simulink model "dual500MHzPFB"  (Simulink 6.2)
settings: Solver=ode45  StartTime=0.0  StopTime=10000  RelTol=1e-3
libraries: xbsIndex_r3 x2070, casper_library x180, xps_library x12, gtkWave x5, gavrt_library x1
(part 10 of 20)

== system dual500MHzPFB/cfgspec/PFB_Subsystem/pfb_fir_real/pol1_in1_last_tap/pfb_real_add_tree ==
  din : Inport  Port=1  LatchInput=off
  sync : Inport  Port=2  LatchInput=off
  Reint0 : xbsIndex_r3/Reinterpret  force_arith_type=on  arith_type="Signed  (2's comp)"  force_bin_pt=on  bin_pt=CoeffBitWidth + BitWidthIn - 2  force_valid=on
  Reint1 : xbsIndex_r3/Reinterpret  force_arith_type=on  arith_type="Signed  (2's comp)"  force_bin_pt=on  bin_pt=CoeffBitWidth + BitWidthIn - 2  force_valid=on
  Slice0 : xbsIndex_r3/Slice  mode=Upper Bit Location + Width  nbits=CoeffBitWidth + BitWidthIn  bit1=-0*(CoeffBitWidth + BitWidthIn)  base1=MSB of Input  bit0=0  base0=MSB of Input  boolean_output=off  explicit_period=off  period=1  dbl_ovrd=off
  Slice1 : xbsIndex_r3/Slice  mode=Upper Bit Location + Width  nbits=CoeffBitWidth + BitWidthIn  bit1=-1*(CoeffBitWidth + BitWidthIn)  base1=MSB of Input  bit0=0  base0=MSB of Input  boolean_output=off  explicit_period=off  period=1  dbl_ovrd=off
  adder_tree1 : Subsystem  AncestorBlock=casper_library/Misc/adder_tree  mask(adder_tree){n_inputs=2, latency=2}
      mask prompts: n_inputs "Number of Inputs"; latency "Add Latency"
      mask help: Sums all inputs using a tree of adds and delays.
      mask init:
      | adder_tree_init(gcb, ...
      |     'n_inputs', n_inputs, ...
      |     'latency', latency);
      settings: AttributesFormatString=latency 2
      mask Help: eval('xlWeb([getenv(''MLIB_ROOT''), ''\doc\html\sp_adder_tree\sp_adder_tree.html''])')
  convert1 : xbsIndex_r3/Convert  arith_type="Signed  (2's comp)"  n_bits=BitWidthOut  bin_pt=BitWidthOut-1  quantization=Truncate  overflow=Saturate  latency=add_latency  explicit_period=off  period=1  dbl_ovrd=off  show_param=off  inserted_by_tool=off  pipeline=off
      settings: xl_area=[0, 0, 0, 0, 0, 0, 0]
  delay1 : xbsIndex_r3/Delay  latency=2  reg_retiming=off  explicit_period=off  period=1  en=off  accept_only_valid=off  init_zero=on  dbl_ovrd=off  show_param=off
      settings: xl_area=[0, 0, 0, 0, 0, 0, 0]
  scale1 : xbsIndex_r3/Scale  scale_factor=-2  explicit_period=off  period=1  dbl_ovrd=off
  dout : Outport
  sync_out : Outport  Port=2
  wires:
  adder_tree1/2(dout) -> scale1/1
  scale1/1 -> convert1/1
  convert1/1 -> dout/1
  sync/1 -> adder_tree1/1(sync)
  adder_tree1/1(sync_out) -> delay1/1
  delay1/1 -> sync_out/1
  din/1 -> Slice0/1, Slice1/1
  Slice0/1 -> Reint0/1
  Reint0/1 -> adder_tree1/2(din1)
  Slice1/1 -> Reint1/1
  Reint1/1 -> adder_tree1/3(din2)

== system dual500MHzPFB/cfgspec/PFB_Subsystem/pfb_fir_real/pol1_in2_first_tap/delay ==
  In1 : Inport  Port=1  LatchInput=off
  delay_bram : casper_library/Delays/delay_bram  DelayLen=2^(PFBSize-n_inputs)  bram_latency=bram_latency
  Out1 : Outport
  wires:
  In1/1 -> delay_bram/1
  delay_bram/1 -> Out1/1

== system dual500MHzPFB/cfgspec/PFB_Subsystem/pfb_fir_real/pol1_in2_first_tap/pfb_coeff_gen ==
  din : Inport  Port=1  LatchInput=off
  sync : Inport  Port=2  LatchInput=off
  Concat : xbsIndex_r3/Concat  num_inputs=2  explicit_period=off  period=1  dbl_ovrd=off
  Counter : xbsIndex_r3/Counter  cnt_type=Free Running  n_bits=8  bin_pt=0  arith_type=Unsigned  start_count=0  cnt_to=Inf  cnt_by_val=1  operation=Up  explicit_period=on  period=1  load_pin=off  rst=on  en=off  dbl_ovrd=off  show_param=off  use_rpm=on  gen_core=off
      settings: xl_area=[0, 0, 0, 0, 0, 0, 0]
  Delay : xbsIndex_r3/Delay  latency=bram_latency+1  reg_retiming=off  explicit_period=off  period=1  en=off  accept_only_valid=off  init_zero=on  dbl_ovrd=off  show_param=off
      settings: xl_area=[0, 0, 0, 0, 0, 0, 0]
  Delay1 : xbsIndex_r3/Delay  latency=3  reg_retiming=off  explicit_period=off  period=1  en=off  accept_only_valid=off  init_zero=on  dbl_ovrd=off  show_param=off
      settings: xl_area=[0, 0, 0, 0, 0, 0, 0]
  ROM1 : xbsIndex_r3/ROM  depth=256  initVector=[7.82033640873917e-005 0.000392792117321438 0.00071082554813207 0.00103311892199487 0.00136049907461725 0.00169380402655518 0.00203388258985642 0.00238159396690193 0.00273780734162119 0.00310340146326166 0.00347926422289714 0.00386629222286377 0.00426539033931678 0.00467747127810509 0.00510345512416486 0.00554426888463693 0.00600084602591724 0.00647412600485223 0.00696505379429587 0.00747457940324748 0.00800365739179369 0.00855324638108065 0.00912430855854599 0.00971780917864314 0.0103347160592936 0.0109759990743052 0.0116426296419981 0.0123355802102817 0.0130558237384286 0.0138043331757953 0.0145820809377384 0.0153900383789824 0.0162291752646908 0.0171004592395002 0.0180048552947743 0.0189433252343389 0.0199168271389599 0.0209263148298273 0.021972737331309 0.0230570383332419 0.0241801556530246 0.0253430206977808 0.0265465579268609 0.0277916843149512 0.0290793088160584 0.0304103318286413 0.0317856446621574 0.0332061290052946 0.0346726563961596 0.0361860876946888 0.0377472725575551 0.0393570489158354 0.0410162424557095 0.0427256661024564 0.0444861195080145 0.046298388542371 0.0481632447890453 0.0500814450449274 0.0520537308247352 0.0540808278703483 0.0561634456652778 0.0583022769545272 0.0604979972700995 0.0627512644624029 0.0650627182378034 0.067432979702574 0.0698626509134837 0.07235231443527 0.0749025329052334 0.0775138486051921 0.0801867830410294 0.082921836530065 0.0857194877964775 0.0885801935750023 0.0915043882231255 0.0944924833419901 0.0975448674062286 0.100661905402931 0.103843938479953 0.107091283603769 0.110404233227058 0.113783054966233 0.117227991289079 0.120739259212706 0.124317050011981 0.127961528938623 0.131672834951122 0.135451080455663 0.139296351058194 0.143208705327813 0.147188174571609 0.151234762621111 0.155348445630488 0.159529171886614 0.163776861631156 0.168091406894782 0.172472671343625 0.176920490138103 0.18143466980421 0.186014988117371 0.190661193998959 0.195373007425566 0.200150119351105 0.204992191641821 0.209898857024285 0.214869719046434 0.219904352051709 0.225002301166354 0.230163082299916 0.235386182158984 0.240671058274206 0.2460171390406 0.251423823771201 0.256890482764031 0.262416457382418 0.26800106014867 0.273643574851073 0.279343256664236 0.285099332282737 0.290911000068066 0.296777430208813 0.302697764894093 0.308671118500132 0.314696577789995 0.320773202126374 0.326900023697389 0.333076047755331 0.339300252868267 0.345571591184427 0.351888988709288 0.358251345595259 0.364657536443868 0.37110641062034 0.377596792580462 0.384127482209607 0.390697255173799 0.397304863282687 0.40394903486429 0.41062847515137 0.417341866679289 0.424087869695195 0.430865122578368 0.437672242271578 0.444507824723272 0.451370445340415 0.458258659451806 0.46517100278169 0.472105991933451 0.479062124883217 0.486037881483159 0.493031723974274 0.50004209750845 0.507067430679598 0.514106136063612 0.521156610766955 0.528217236983621 0.535286382560249 0.542362401569151 0.549443634889005 0.556528410792964 0.563615045543947 0.570701843996833 0.577787100207321 0.584869098047179 0.591946111825632 0.599016406916601 0.606078240391542 0.613129861657594 0.620169513100771 0.627195430733905 0.634205844849072 0.641198980674199 0.648173059033581 0.655126297012004 0.662056908622189 0.668963105475262 0.675843097453958 0.682695093388247 0.6895173017331 0.696307931248092 0.703065191678525 0.709787294437785 0.716472453290627 0.723118885037072 0.729724810196624 0.736288453692496 0.742808045535534 0.749281821507542 0.755708023843698 0.762084901913749 0.768410712901686 0.774683722483594 0.780902205503364 0.787064446645969 0.793168741108002 0.799213395265163 0.805196727336407 0.811117068044443 0.816972761272283 0.822762164715558 0.828483650530292 0.834135605975834 0.839716434052685 0.84522455413489 0.850658402596745 0.856016433433509 0.861297118875845 0.866498949997721 0.871620437317469 0.876660111391761 0.881616523402199 0.886488245734271 0.891273872548405 0.89597202034285 0.900581328508143 0.905100459872888 0.909528101240623 ...(+701 chars)]  arith_type="Signed  (2's comp)"  n_bits=8  bin_pt=7  latency=2  init_zero=on  explicit_period=off  period=1  rst=off  init_reg=0  en=off  dbl_ovrd=off  show_param=on  distributed_mem=off  use_rpm=on  gen_core=off
      settings: xl_area=[0, 0, 0, 0, 0, 0, 0]
  ROM2 : xbsIndex_r3/ROM  depth=256  initVector=[0.999993555614484 0.999895235614821 0.999677407720508 0.999340137306542 0.99888352558091 0.998307709543272 0.997612861929031 0.996799191138817 0.995866941153415 0.994816391434173 0.993647856808947 0.992361687343622 0.99095826819928 0.989438019475073 0.987801396036875 0.986048887331801 0.984181017188665 0.982198343604478 0.980101458517079 0.977890987564016 0.975567589827767 0.973131957567446 0.970584815937088 0.967926922690669 0.965159067873983 0.962282073503518 0.959296793232491 0.956204112004174 0.953004945692698 0.949700240731477 0.946290973729442 0.942778151075241 0.939162808529609 0.935446010806083 0.931628851140254 0.927712450847762 0.923697958871232 0.919586551316358 0.915379430977356 0.911077826851989 0.906682993646407 0.902196211270012 0.897618784320587 0.892952041559925 0.888197335380202 0.883356041261322 0.878429557219512 0.873419303247388 0.868326720745771 0.863153271947495 0.857900439333497 0.852569725041413 0.847162650267003 0.841680754658628 0.83612559570509 0.830498748117097 0.824801803202644 0.819036368236582 0.813204065824676 0.807306533262431 0.801345421888981 0.795322396436338 0.789239134374282 0.783097325251212 0.776898670031231 0.770644880427786 0.764337678234152 0.757978794651064 0.751569969611804 0.745112951105048 0.738609494495772 0.732061361844525 0.725470321225382 0.718838146042869 0.71216661434818 0.705457508154989 0.698712612755152 0.691933716034627 0.685122607789892 0.678281079045185 0.671410921370864 0.66451392620319 0.657591884165825 0.65064658439337 0.643679813857221 0.636693356694045 0.629688993537183 0.622668500851263 0.615633650270321 0.608586207939725 0.601527933862177 0.594460581248096 0.587385895870655 0.580305615425757 0.573221468897224 0.566135175927489 0.55904844619404 0.551962978791909 0.544880461622458 0.537802570788727 0.530730969997615 0.52366730996913 0.516613227852975 0.509570346652719 0.502540274657783 0.495524604883502 0.488524914519479 0.481542764386477 0.474579698402069 0.467637243055272 0.460716906890385 0.453820180000238 0.446948533529066 0.440103419185214 0.433286268763866 0.426498493679995 0.419741484511721 0.413016610554267 0.406325219384677 0.399668636437484 0.393048164591489 0.386465083767804 0.379920650539333 0.373416097751825 0.366952634156649 0.360531444055436 0.354153686956706 0.347820497244626 0.34153298386 0.335292229993622 0.329099292792089 0.322955203076182 0.316860965071917 0.310817556154338 0.304825926604156 0.2988869993773 0.293001669887455 0.287170805801649 0.281395246848952 0.275675804642333 0.270013262513728 0.264408375362351 0.258861869516288 0.253374442607394 0.247946763459516 0.242579471990057 0.237273179124887 0.232028466726598 0.226845887536105 0.221725965127573 0.21666919387666 0.211676038942041 0.206746936260191 0.201882292553387 0.197082485350882 0.192347863023202 0.187678744829518 0.183075420978016 0.178538152699211 0.174067172332122 0.169662683423225 0.165324860838114 0.161053850885749 0.156849771455227 0.152712712164937 0.148642734524024 0.144639872106008 0.14070413073448 0.136835488680706 0.133033896873036 0.129299279117972 0.125631532332744 0.12203052678926 0.118496106369262 0.115028088830537 0.111626266084031 0.108290404481666 0.105020245114723 0.101815504122587 0.0986758730116877 0.0956010189844369 0.0925905852779795 0.0896441915125591 0.0867614340492978 0.0839418863571882 0.0811850993890874 0.0784906019665026 0.0758579011729519 0.0732864827556818 0.0707758115355173 0.0683253318246198 0.0659344678519223 0.0636026241960095 0.0613291862252073 0.0591135205446423 0.056954975450031 0.0548528813879534 0.0528065514223651 0.0508152817070987 0.0488783519641021 0.0469950259671621 0.0451645520308558 0.0433861635044739 0.0416590792706549 0.0399825042484717 0.0383556299007058 0.0367776347450473 0.0352476848689546 0.0337649344479084 0.0323285262667932 0.0309375922441371 0.029591253958944 0.0282886231798464 0.0270288023963116 0.0258108853516301 0.0246339575774173 0.0234970969293587 0.0223993741239277 0.0213398532758088 0.0203175924357544 ...(+708 chars)]  arith_type="Signed  (2's comp)"  n_bits=8  bin_pt=7  latency=2  init_zero=on  explicit_period=off  period=1  rst=off  init_reg=0  en=off  dbl_ovrd=off  show_param=on  distributed_mem=off  use_rpm=on  gen_core=off
      settings: xl_area=[0, 0, 0, 0, 0, 0, 0]
  Register : xbsIndex_r3/Register  init=0  reg_only_valid=off  explicit_period=off  period=1  rst=off  en=off  out_en=off  dbl_ovrd=off  show_param=off
      settings: xl_area=[0, 0, 0, 0, 0, 0, 0]
  Reinterpret1 : xbsIndex_r3/Reinterpret  force_arith_type=on  arith_type=Unsigned  force_bin_pt=on  bin_pt=0  force_valid=on
  Reinterpret2 : xbsIndex_r3/Reinterpret  force_arith_type=on  arith_type=Unsigned  force_bin_pt=on  bin_pt=0  force_valid=on
  dout : Outport
  sync_out : Outport  Port=2
  coeff : Outport  Port=3
  wires:
  din/1 -> Delay1/1
  Delay1/1 -> dout/1
  sync/1 -> Counter/1, Delay/1
  Delay/1 -> sync_out/1
  Concat/1 -> Register/1
  Register/1 -> coeff/1
  Counter/1 -> ROM1/1, ROM2/1
  ROM1/1 -> Reinterpret1/1
  Reinterpret1/1 -> Concat/1
  ROM2/1 -> Reinterpret2/1
  Reinterpret2/1 -> Concat/2

== system dual500MHzPFB/cfgspec/PFB_Subsystem/pfb_fir_real/pol1_in2_last_tap/pfb_real_add_tree ==
  din : Inport  Port=1  LatchInput=off
  sync : Inport  Port=2  LatchInput=off
  Reint0 : xbsIndex_r3/Reinterpret  force_arith_type=on  arith_type="Signed  (2's comp)"  force_bin_pt=on  bin_pt=CoeffBitWidth + BitWidthIn - 2  force_valid=on
  Reint1 : xbsIndex_r3/Reinterpret  force_arith_type=on  arith_type="Signed  (2's comp)"  force_bin_pt=on  bin_pt=CoeffBitWidth + BitWidthIn - 2  force_valid=on
  Slice0 : xbsIndex_r3/Slice  mode=Upper Bit Location + Width  nbits=CoeffBitWidth + BitWidthIn  bit1=-0*(CoeffBitWidth + BitWidthIn)  base1=MSB of Input  bit0=0  base0=MSB of Input  boolean_output=off  explicit_period=off  period=1  dbl_ovrd=off
  Slice1 : xbsIndex_r3/Slice  mode=Upper Bit Location + Width  nbits=CoeffBitWidth + BitWidthIn  bit1=-1*(CoeffBitWidth + BitWidthIn)  base1=MSB of Input  bit0=0  base0=MSB of Input  boolean_output=off  explicit_period=off  period=1  dbl_ovrd=off
  adder_tree1 : Subsystem  AncestorBlock=casper_library/Misc/adder_tree  mask(adder_tree){n_inputs=2, latency=2}
      mask prompts: n_inputs "Number of Inputs"; latency "Add Latency"
      mask help: Sums all inputs using a tree of adds and delays.
      mask init:
      | adder_tree_init(gcb, ...
      |     'n_inputs', n_inputs, ...
      |     'latency', latency);
      settings: AttributesFormatString=latency 2
      mask Help: eval('xlWeb([getenv(''MLIB_ROOT''), ''\doc\html\sp_adder_tree\sp_adder_tree.html''])')
  convert1 : xbsIndex_r3/Convert  arith_type="Signed  (2's comp)"  n_bits=BitWidthOut  bin_pt=BitWidthOut-1  quantization=Truncate  overflow=Saturate  latency=add_latency  explicit_period=off  period=1  dbl_ovrd=off  show_param=off  inserted_by_tool=off  pipeline=off
      settings: xl_area=[0, 0, 0, 0, 0, 0, 0]
  delay1 : xbsIndex_r3/Delay  latency=2  reg_retiming=off  explicit_period=off  period=1  en=off  accept_only_valid=off  init_zero=on  dbl_ovrd=off  show_param=off
      settings: xl_area=[0, 0, 0, 0, 0, 0, 0]
  scale1 : xbsIndex_r3/Scale  scale_factor=-2  explicit_period=off  period=1  dbl_ovrd=off
  dout : Outport
  sync_out : Outport  Port=2
  wires:
  adder_tree1/2(dout) -> scale1/1
  scale1/1 -> convert1/1
  convert1/1 -> dout/1
  sync/1 -> adder_tree1/1(sync)
  adder_tree1/1(sync_out) -> delay1/1
  delay1/1 -> sync_out/1
  din/1 -> Slice0/1, Slice1/1
  Slice0/1 -> Reint0/1
  Reint0/1 -> adder_tree1/2(din1)
  Slice1/1 -> Reint1/1
  Reint1/1 -> adder_tree1/3(din2)

== system dual500MHzPFB/cfgspec/PFB_Subsystem/pfb_fir_real/pol1_in3_first_tap/delay ==
  In1 : Inport  Port=1  LatchInput=off
  delay_bram : casper_library/Delays/delay_bram  DelayLen=2^(PFBSize-n_inputs)  bram_latency=bram_latency
  Out1 : Outport
  wires:
  In1/1 -> delay_bram/1
  delay_bram/1 -> Out1/1

== system dual500MHzPFB/cfgspec/PFB_Subsystem/pfb_fir_real/pol1_in3_first_tap/pfb_coeff_gen ==
  din : Inport  Port=1  LatchInput=off
  sync : Inport  Port=2  LatchInput=off
  Concat : xbsIndex_r3/Concat  num_inputs=2  explicit_period=off  period=1  dbl_ovrd=off
  Counter : xbsIndex_r3/Counter  cnt_type=Free Running  n_bits=8  bin_pt=0  arith_type=Unsigned  start_count=0  cnt_to=Inf  cnt_by_val=1  operation=Up  explicit_period=on  period=1  load_pin=off  rst=on  en=off  dbl_ovrd=off  show_param=off  use_rpm=on  gen_core=off
      settings: xl_area=[0, 0, 0, 0, 0, 0, 0]
  Delay : xbsIndex_r3/Delay  latency=bram_latency+1  reg_retiming=off  explicit_period=off  period=1  en=off  accept_only_valid=off  init_zero=on  dbl_ovrd=off  show_param=off
      settings: xl_area=[0, 0, 0, 0, 0, 0, 0]
  Delay1 : xbsIndex_r3/Delay  latency=3  reg_retiming=off  explicit_period=off  period=1  en=off  accept_only_valid=off  init_zero=on  dbl_ovrd=off  show_param=off
      settings: xl_area=[0, 0, 0, 0, 0, 0, 0]
  ROM1 : xbsIndex_r3/ROM  depth=256  initVector=[0.000156571753004131 0.000471945891501983 0.000790967418464927 0.00111445452761384 0.00144323688731232 0.0017781552531742 0.00212006107274008 0.0024698160823956 0.00282829189670815 0.00319636959036365 0.00357493927288892 0.00396489965634961 0.00436715761621773 0.00478262774560706 0.00521223190307826 0.00565689875421988 0.00611756330721485 0.006595166442606 0.0070906544374775 0.00760497848427273 0.00813909420447243 0.00869396115736018 0.00927054234410557 0.00986980370739833 0.0104927136268696 0.0111402424105394 0.0118133617825326 0.0125130443673066 0.0132402631706387 0.013995991057622 0.0147812002279213 0.0155968616885416 0.016443944724367 0.0173234163667243 0.0182362408602338 0.0191833791282049 0.0201657882368408 0.0211844208585156 0.0222402247343869 0.0233341421366126 0.0244671093304362 0.0256400560364093 0.0268539048930204 0.028109570919997 0.0294079609825521 0.0307499732568442 0.0321364966969199 0.0335684105034094 0.0350465835942454 0.0365718740776727 0.03814512872782 0.0397671824631001 0.0414388578277084 0.0431609644764848 0.0449342986634068 0.0467596427339775 0.0486377646217729 0.0505694173494113 0.0525553385342047 0.0545962498987528 0.0566928567867364 0.0588458476841667 0.0610558937463428 0.0633236483307712 0.0656497465362942 0.0680348047486762 0.0704794201928911 0.0729841704923531 0.0755496132353287 0.0781762855487681 0.080864703679787 0.0836153625850295 0.0864287355281387 0.0893052736855576 0.0922454057608818 0.0952495376079764 0.0983180518630736 0.101451307586057 0.104649639911135 0.107913359707113 0.111242753247444 0.114638081890267 0.118099581768609 0.121627463490941 0.125221911852256 0.128883085555861 0.132611116946024 0.136406111751676 0.140268148841289 0.144197279989117 0.148193529652922 0.152256894763353 0.156387344525091 0.160584820229917 0.164849235081815 0.169180474034232 0.173578393639624 0.178042821911379 0.182573558198244 0.187170373071336 0.191833008223839 0.196561176383476 0.201354561237828 0.206212817372591 0.211135570222817 0.216122416037231 0.22117292185565 0.226286625499582 0.231463035576027 0.236701631494537 0.242001863497553 0.247363152704048 0.252784891166504 0.258266441941216 0.263807139171958 0.269406288186976 0.275063165609337 0.280777019480592 0.286547069397754 0.292372506663552 0.298252494449934 0.304186167974785 0.310172634691807 0.316210974493512 0.322300239927273 0.328439456424369 0.334627622541945 0.340863710217824 0.347146665038078 0.353475406517269 0.359848828391271 0.36626579892256 0.372725161217884 0.379225733558168 0.385766309740569 0.392345659432526 0.398962528537691 0.405615639573596 0.412303692060908 0.419025362924137 0.425779306903621 0.432564156978649 0.439378524801535 0.446221001142489 0.453090156345094 0.459984540792213 0.466902685382136 0.473843102014779 0.48080428408772 0.487784707001898 0.49478282867673 0.501797090074468 0.508825915733558 0.515867714310774 0.522920879131923 0.529983788750869 0.537054807516645 0.54413228614842 0.551214562318069 0.558299961240106 0.565386796268718 0.572473369501655 0.579557972390709 0.586638886358525 0.593714383421474 0.600782726818319 0.607842171644411 0.614890965491117 0.62192734909023 0.628949556963061 0.635955818073934 0.642944356487798 0.649913392031675 0.656861140959638 0.663785816621042 0.670685630131702 0.677558791047733 0.684403508041737 0.691217989581062 0.698000444607801 0.704749083220269 0.711462117355605 0.718137761473247 0.724774233238938 0.731369754208968 0.737922550514358 0.744430853544664 0.750892900631098 0.757306935728673 0.763671210097042 0.769983982979752 0.776243522281579 0.782448105243668 0.788596019116149 0.794685561827938 0.800715042653424 0.806682782875726 0.812587116446239 0.818426390640147 0.824198966707636 0.829903220520478 0.835537543213724 0.84110034182219 0.846590039911459 0.852005078203117 0.85734391519392 0.862605027768629 0.867786911806227 0.872888082779229 0.87790707634584 0.88284244893466 0.887692778321693 0.892456664199373 0.897132728737377 0.901719617134936 0.90621599816441 0.910620564705884 ...(+696 chars)]  arith_type="Signed  (2's comp)"  n_bits=8  bin_pt=7  latency=2  init_zero=on  explicit_period=off  period=1  rst=off  init_reg=0  en=off  dbl_ovrd=off  show_param=on  distributed_mem=off  use_rpm=on  gen_core=off
      settings: xl_area=[0, 0, 0, 0, 0, 0, 0]
  ROM2 : xbsIndex_r3/ROM  depth=256  initVector=[0.999980181706812 0.999851980565338 0.999604284511911 0.999237167882849 0.998750740838502 0.998145149318279 0.99742057498107 0.996577235131088 0.995615382629159 0.994535305789518 0.993337328262134 0.99202180890064 0.990589141615924 0.989039755215435 0.987374113228298 0.985592713716306 0.983696089070883 0.981684805796099 0.979559464277863 0.97732069853937 0.974969175982937 0.972505597118337 0.969930695277763 0.967245236317542 0.96445001830675 0.961545871202867 0.958533656514614 0.955414266952141 0.952188626064713 0.948857687866076 0.945422436447659 0.941883885579808 0.938243078301218 0.934501086496762 0.93065901046392 0.926717978467979 0.922679146286243 0.918543696741437 0.914312839224529 0.909987809207196 0.905569867744142 0.901060300965507 0.896460419559603 0.891771558246203 0.886995075240635 0.882132351708915 0.877184791214188 0.872153819154706 0.867040882193617 0.86184744768082 0.856575003067155 0.851225055311182 0.845799130278843 0.840298772136253 0.83472554273592 0.829081020996665 0.823366802277519 0.817584497745891 0.811735733740289 0.805822151127884 0.799845404657212 0.793807162306308 0.787709104626554 0.781552924082562 0.775340324388371 0.76907301984027 0.762752734646535 0.756381202254406 0.749960164674578 0.743491371803535 0.736976580744021 0.730417555123955 0.723816064414095 0.71717388324476 0.710492790721915 0.703774569742931 0.697021006312307 0.690233888857689 0.683415007546466 0.676566153603261 0.669689118628614 0.662785693919171 0.655857669789663 0.648906834896993 0.641934975566721 0.634943875122243 0.627935313216969 0.620911065169787 0.613872901304108 0.606822586290777 0.599761878495151 0.592692529328615 0.585616282604827 0.578534873900973 0.571450029924306 0.56436346788425 0.557276894870328 0.550192007236204 0.543110489990084 0.536034016191747 0.528964246356468 0.521902827866082 0.514851394387443 0.507811565298521 0.500784945122391 0.493773122969342 0.486777671987345 0.479800148821113 0.472842093079979 0.465905026814805 0.458990454004159 0.452099860049946 0.445234711282726 0.438396454476901 0.431586516375986 0.424806303228137 0.418057200332153 0.411340571594091 0.40465775909472 0.398010082667942 0.391398839490374 0.384825303682239 0.378290725919721 0.371796333058942 0.365343327771685 0.358932888193021 0.352566167580962 0.34624429398826 0.33996836994648 0.333739472162456 0.32755865122724 0.321426931337641 0.31534531003045 0.309314757929439 0.303336218505222 0.297410607848047 0.291538814453586 0.2857216990218 0.279960094268917 0.274254804752596 0.268606606710293 0.263016247910897 0.257484447519645 0.252011895976347 0.246599254886948 0.241247156928422 0.235956205767024 0.230726975989882 0.225560013049927 0.220455833224157 0.215414923585196 0.210437741986143 0.205524717058656 0.20067624822426 0.195892705718796 0.191174430630003 0.18652173494814 0.181934901629597 0.177414184673436 0.172959809210765 0.168571971606878 0.164250839576072 0.159996552309034 0.155809220612716 0.151688927062585 0.147635726167125 0.143649644544501 0.139730681111232 0.135878807282765 0.132093967185811 0.128376077882305 0.124725029604834 0.121140686003409 0.117622884403397 0.114171436074477 0.110786126510436 0.107466715719658 0.104212938526102 0.101024504880621 0.0979011001824149 0.0948423856104419 0.0918479984645913 0.088917552516421 0.0860506383692603 0.083246823827471 0.0805056542746607 0.0778266530606313 0.0752093218968506 0.0726531412602235 0.0701575708049404 0.0677220497821762 0.0653459974674089 0.0630288135951235 0.0607698788006672 0.0585685550690139 0.0564241861901975 0.054336098221168 0.0523035999538251 0.0503259833889764 0.048402524215972 0.0465324822977585 0.0447151021610977 0.0429496134916917 0.0412352316339554 0.0395711580951738 0.0379565810537831 0.0363906758715103 0.0348726056091064 0.0334015215454071 0.0319765636994546 0.0305968613554102 0.0292615335899919 0.0279696898021663 0.0267204302448249 0.0255128465581769 0.0243460223045864 0.0232190335045865 0.0221309491737983 0.0210808318604881 0.0200677381834912 0.0190907193702359 ...(+687 chars)]  arith_type="Signed  (2's comp)"  n_bits=8  bin_pt=7  latency=2  init_zero=on  explicit_period=off  period=1  rst=off  init_reg=0  en=off  dbl_ovrd=off  show_param=on  distributed_mem=off  use_rpm=on  gen_core=off
      settings: xl_area=[0, 0, 0, 0, 0, 0, 0]
  Register : xbsIndex_r3/Register  init=0  reg_only_valid=off  explicit_period=off  period=1  rst=off  en=off  out_en=off  dbl_ovrd=off  show_param=off
      settings: xl_area=[0, 0, 0, 0, 0, 0, 0]
  Reinterpret1 : xbsIndex_r3/Reinterpret  force_arith_type=on  arith_type=Unsigned  force_bin_pt=on  bin_pt=0  force_valid=on
  Reinterpret2 : xbsIndex_r3/Reinterpret  force_arith_type=on  arith_type=Unsigned  force_bin_pt=on  bin_pt=0  force_valid=on
  dout : Outport
  sync_out : Outport  Port=2
  coeff : Outport  Port=3
  wires:
  din/1 -> Delay1/1
  Delay1/1 -> dout/1
  sync/1 -> Counter/1, Delay/1
  Delay/1 -> sync_out/1
  Concat/1 -> Register/1
  Register/1 -> coeff/1
  Counter/1 -> ROM1/1, ROM2/1
  ROM1/1 -> Reinterpret1/1
  Reinterpret1/1 -> Concat/1
  ROM2/1 -> Reinterpret2/1
  Reinterpret2/1 -> Concat/2

== system dual500MHzPFB/cfgspec/PFB_Subsystem/pfb_fir_real/pol1_in3_last_tap/pfb_real_add_tree ==
  din : Inport  Port=1  LatchInput=off
  sync : Inport  Port=2  LatchInput=off
  Reint0 : xbsIndex_r3/Reinterpret  force_arith_type=on  arith_type="Signed  (2's comp)"  force_bin_pt=on  bin_pt=CoeffBitWidth + BitWidthIn - 2  force_valid=on
  Reint1 : xbsIndex_r3/Reinterpret  force_arith_type=on  arith_type="Signed  (2's comp)"  force_bin_pt=on  bin_pt=CoeffBitWidth + BitWidthIn - 2  force_valid=on
  Slice0 : xbsIndex_r3/Slice  mode=Upper Bit Location + Width  nbits=CoeffBitWidth + BitWidthIn  bit1=-0*(CoeffBitWidth + BitWidthIn)  base1=MSB of Input  bit0=0  base0=MSB of Input  boolean_output=off  explicit_period=off  period=1  dbl_ovrd=off
  Slice1 : xbsIndex_r3/Slice  mode=Upper Bit Location + Width  nbits=CoeffBitWidth + BitWidthIn  bit1=-1*(CoeffBitWidth + BitWidthIn)  base1=MSB of Input  bit0=0  base0=MSB of Input  boolean_output=off  explicit_period=off  period=1  dbl_ovrd=off
  adder_tree1 : Subsystem  AncestorBlock=casper_library/Misc/adder_tree  mask(adder_tree){n_inputs=2, latency=2}
      mask prompts: n_inputs "Number of Inputs"; latency "Add Latency"
      mask help: Sums all inputs using a tree of adds and delays.
      mask init:
      | adder_tree_init(gcb, ...
      |     'n_inputs', n_inputs, ...
      |     'latency', latency);
      settings: AttributesFormatString=latency 2
      mask Help: eval('xlWeb([getenv(''MLIB_ROOT''), ''\doc\html\sp_adder_tree\sp_adder_tree.html''])')
  convert1 : xbsIndex_r3/Convert  arith_type="Signed  (2's comp)"  n_bits=BitWidthOut  bin_pt=BitWidthOut-1  quantization=Truncate  overflow=Saturate  latency=add_latency  explicit_period=off  period=1  dbl_ovrd=off  show_param=off  inserted_by_tool=off  pipeline=off
      settings: xl_area=[0, 0, 0, 0, 0, 0, 0]
  delay1 : xbsIndex_r3/Delay  latency=2  reg_retiming=off  explicit_period=off  period=1  en=off  accept_only_valid=off  init_zero=on  dbl_ovrd=off  show_param=off
      settings: xl_area=[0, 0, 0, 0, 0, 0, 0]
  scale1 : xbsIndex_r3/Scale  scale_factor=-2  explicit_period=off  period=1  dbl_ovrd=off
  dout : Outport
  sync_out : Outport  Port=2
  wires:
  adder_tree1/2(dout) -> scale1/1
  scale1/1 -> convert1/1
  convert1/1 -> dout/1
  sync/1 -> adder_tree1/1(sync)
  adder_tree1/1(sync_out) -> delay1/1
  delay1/1 -> sync_out/1
  din/1 -> Slice0/1, Slice1/1
  Slice0/1 -> Reint0/1
  Reint0/1 -> adder_tree1/2(din1)
  Slice1/1 -> Reint1/1
  Reint1/1 -> adder_tree1/3(din2)

== system dual500MHzPFB/cfgspec/PFB_Subsystem/pfb_fir_real/pol1_in4_first_tap/delay ==
  In1 : Inport  Port=1  LatchInput=off
  delay_bram : casper_library/Delays/delay_bram  DelayLen=2^(PFBSize-n_inputs)  bram_latency=bram_latency
  Out1 : Outport
  wires:
  In1/1 -> delay_bram/1
  delay_bram/1 -> Out1/1

== system dual500MHzPFB/cfgspec/PFB_Subsystem/pfb_fir_real/pol1_in4_first_tap/pfb_coeff_gen ==
  din : Inport  Port=1  LatchInput=off
  sync : Inport  Port=2  LatchInput=off
  Concat : xbsIndex_r3/Concat  num_inputs=2  explicit_period=off  period=1  dbl_ovrd=off
  Counter : xbsIndex_r3/Counter  cnt_type=Free Running  n_bits=8  bin_pt=0  arith_type=Unsigned  start_count=0  cnt_to=Inf  cnt_by_val=1  operation=Up  explicit_period=on  period=1  load_pin=off  rst=on  en=off  dbl_ovrd=off  show_param=off  use_rpm=on  gen_core=off
      settings: xl_area=[0, 0, 0, 0, 0, 0, 0]
  Delay : xbsIndex_r3/Delay  latency=bram_latency+1  reg_retiming=off  explicit_period=off  period=1  en=off  accept_only_valid=off  init_zero=on  dbl_ovrd=off  show_param=off
      settings: xl_area=[0, 0, 0, 0, 0, 0, 0]
  Delay1 : xbsIndex_r3/Delay  latency=3  reg_retiming=off  explicit_period=off  period=1  en=off  accept_only_valid=off  init_zero=on  dbl_ovrd=off  show_param=off
      settings: xl_area=[0, 0, 0, 0, 0, 0, 0]
  ROM1 : xbsIndex_r3/ROM  depth=256  initVector=[0.000235117647765776 0.000551327569575741 0.000871388331650675 0.00119612103225011 0.00152635814818096 0.00186294314540636 0.0022067300817663 0.00255858320198372 0.00291937652513412 0.00328999342476105 0.00367132620182454 0.00406427565067298 0.00446975061823393 0.00488866755662283 0.00532195006937266 0.00577052845149145 0.00623533922355848 0.00671732466007321 0.00721743231227507 0.00773661452565523 0.00827582795238525 0.00883603305889021 0.00941819362879768 0.0100232762614963 0.0106522498665412 0.0113060851541457 0.0119857541220021 0.0126922295386765 0.0134264844238244 0.0141894915254781 0.0149822227946568 0.0158056488575538 0.0166607384855574 0.017548458063362 0.0184697710554301 0.0194256374710662 0.0204170133283646 0.0214448501172952 0.0225100942621926 0.0236136865839149 0.0247565617619379 0.0259396477966543 0.0271638654721455 0.0284301278196944 0.0297393395823103 0.031092396680534 0.0324901856797932 0.0339335832595792 0.0354234556847124 0.0369606582789679 0.0385460349013288 0.0401804174251365 0.0418646252204042 0.0435994646395624 0.0453857285069007 0.0472241956119709 0.0491156302072151 0.0510607815100817 0.0530603832098875 0.0551151529796884 0.0572257919934118 0.0593929844485101 0.0616173970943848 0.0638996787668347 0.0662404599287766 0.0686403522174832 0.071099947998584 0.0736198199270695 0.0762005205155353 0.0788425817099054 0.0815465144728618 0.0843128083752139 0.0871419311954306 0.0900343285275589 0.092990423397747 0.0960106158895877 0.0990952827784922 0.102244777175303 0.105459428179349 0.108739540541143 0.112085394334912 0.115497244641159 0.118975321239438 0.12251982831152 0.126130944155138 0.129808820908474 0.133553584285556 0.13736533332274 0.141244140136412 0.145190049692087 0.149203079585039 0.153283219832602 0.157430432678291 0.161644652407862 0.165925785177441 0.170273708853853 0.174688272867243 0.179169298076123 0.183716576644931 0.188329871934205 0.193008918403472 0.197753421526913 0.202563057721923 0.207437474290597 0.212376289374241 0.217379091920954 0.222445441666344 0.227574869127416 0.232766875609693 0.238020933227584 0.243336484938052 0.248712944587585 0.254149696972505 0.259646097912613 0.265201474338185 0.270815124390307 0.276486317534554 0.282214294687982 0.287998268359427 0.293837422803077 0.299730914185284 0.305677870764572 0.311677393084804 0.317728554181443 0.323830399800861 0.329981948632614 0.336182192554631 0.342430096891214 0.348724600683793 0.355064616974316 0.361449033101202 0.367876711007733 0.374346487562795 0.380857174893835 0.38740756073192 0.393996408768776 0.400622459025663 0.407284428233955 0.41398101022727 0.420710876345013 0.427472675847161 0.434265036340141 0.441086564213617 0.44793584508803 0.454811444272702 0.461711907234316 0.468635760075602 0.475581510024006 0.482547645930165 0.489532638775981 0.496534942192067 0.503552992984374 0.510585211669765 0.517630003020315 0.524685756616119 0.531750847406352 0.538823636278379 0.545902470634637 0.552985684977073 0.560071601498875 0.567158530683245 0.574244771908958 0.581328614062453 0.588408336156179 0.59548220795295 0.60254849059601 0.609605437244566 0.616651293714493 0.623684299123933 0.63070268654352 0.637704683650928 0.644688513389471 0.651652394630459 0.65859454283902 0.665513170743091 0.672406489005293 0.679272706897384 0.686110032976994 0.692916675766342 0.699690844432641 0.706430749469876 0.713134603381663 0.719800621364874 0.726427021993738 0.733012027904095 0.739553866477515 0.746050770524958 0.752500978969682 0.758902737529087 0.76525429939519 0.771553925913424 0.777799887259458 0.783990463113728 0.790123943333386 0.796198628621342 0.802212831192126 0.808164875434248 0.814053098568757 0.819875851303714 0.825631498484268 0.831318419738052 0.836935010115596 0.842479680725471 0.84795085936388 0.853346991138395 0.858666539085575 0.863907984782168 0.869069828949628 0.874150592051666 0.879148814884566 0.884063059159991 0.888891908080022 0.893633966904157 0.898287863508018 0.902852248933504 0.907325797930147 0.911707209487413 ...(+699 chars)]  arith_type="Signed  (2's comp)"  n_bits=8  bin_pt=7  latency=2  init_zero=on  explicit_period=off  period=1  rst=off  init_reg=0  en=off  dbl_ovrd=off  show_param=on  distributed_mem=off  use_rpm=on  gen_core=off
      settings: xl_area=[0, 0, 0, 0, 0, 0, 0]
  ROM2 : xbsIndex_r3/ROM  depth=256  initVector=[0.999959336786865 0.999801256908778 0.999523697342405 0.999126741383489 0.998610508141931 0.997975152493165 0.997220865014935 0.99634787190949 0.99535643491125 0.994246851179977 0.993019453179501 0.991674608542054 0.990212719918283 0.988634224813006 0.986939595406783 0.985129338363398 0.983203994623318 0.981164139183251 0.979010380861888 0.976743362051936 0.974363758458571 0.971872278824412 0.969269664641163 0.96655668984804 0.963734160517132 0.960802914525833 0.957763821216508 0.954617781043538 0.951365725207906 0.948008615279514 0.944547442807368 0.940983228917847 0.937317023901219 0.933549906786599 0.92968298490555 0.92571739344452 0.921654294986329 0.917494879040905 0.913240361565502 0.908891984474602 0.904451015139734 0.899918745879451 0.895296493439671 0.890585598464651 0.885787424958816 0.880903359739698 0.875934811882229 0.870883212154659 0.865750012446327 0.860536685187583 0.855244722762093 0.849875636911818 0.844430958134928 0.838912235076933 0.833321033915289 0.827658937737797 0.821927545915033 0.816128473467133 0.810263350425193 0.804333821187595 0.798341543871533 0.792288189660053 0.78617544214488 0.780004996665351 0.773778559643742 0.767497847917287 0.761164588067204 0.754780515745012 0.748347374996464 0.741866917583381 0.735340902303706 0.72877109431008 0.722159264427236 0.715507188468543 0.70881664655197 0.702089422415814 0.695327302734468 0.688532076434552 0.681705534011708 0.674849466848357 0.667965666532734 0.661055924179494 0.654122029752188 0.647165771387927 0.640188934724505 0.633193302230307 0.62618065253728 0.619152759777259 0.612111392921958 0.605058315126893 0.597995283079545 0.590924046352026 0.583846346758558 0.576763917718018 0.569678483621844 0.562591759207569 0.555505448938255 0.548421246388095 0.541340833634453 0.53426588065659 0.527198044741348 0.520138969896043 0.513090286268806 0.506053609576635 0.499030540541388 0.492022664333961 0.485031550026882 0.478058750055559 0.471105799688386 0.464174216505958 0.457265499889588 0.450381130519337 0.443522569881787 0.436691259787727 0.42988862189997 0.423116057271485 0.41637494589403 0.409666646257468 0.40299249491994 0.396353806089064 0.389751871214329 0.383187958590841 0.376663312974563 0.37017915520922 0.363736681864985 0.3573370648891 0.350981451268552 0.344670962704932 0.338406695301595 0.332189719263226 0.326021078607927 0.31990179089192 0.31383284694696 0.30781521063054 0.301849818588976 0.295937580033444 0.290079376529033 0.284276061796883 0.278528461529458 0.272837373218999 0.267203565999214 0.261627780500222 0.256110728716798 0.250653093889933 0.245255530401722 0.239918663683604 0.234643090137943 0.229429377072959 0.224278062650994 0.219189655850098 0.214164636438918 0.209203454964854 0.204306532755457 0.199474261933023 0.194707005442337 0.190005097091513 0.18536884160587 0.180798514694791 0.176294363131469 0.171856604845487 0.167485429028132 0.163180996250367 0.158943438593346 0.154772859791397 0.15066933538734 0.146632912900048 0.142663612004118 0.138761424721536 0.134926315625203 0.131158222054187 0.12745705434057 0.123822696047722 0.120255004219878 0.116753809642842 0.113318917115668 0.109950105733148 0.106647129178934 0.103409716029124 0.100237570066129 0.0971303706026347 0.0940877728154699 0.0911094080891901 0.0881948843691749 0.0853437865240404 0.0825556767171574 0.0798300947870689 0.07716655863659 0.0745645646303748 0.0720235880007281 0.0695430832614382 0.0671224846294021 0.0647612064538125 0.0624586436526723 0.0602141721563989 0.0580271493582791 0.0558969145715315 0.0538227894927295 0.0518040786713401 0.049840069985125 0.0479300351211532 0.0460732300621711 0.0442688955780716 0.0425162577222057 0.0408145283322752 0.0391629055355467 0.0375605742581208 0.036006706737996 0.0345004630416585 0.033040991583933 0.0316274296508277 0.0302589039251033 0.028934531014299 0.0276534179809465 0.0264146628746999 0.0252173552661157 0.024060576781809 0.0229434016407191 0.0218648971912137 0.0208241244487622 0.0198201386339105 0.0188519897102879 ...(+691 chars)]  arith_type="Signed  (2's comp)"  n_bits=8  bin_pt=7  latency=2  init_zero=on  explicit_period=off  period=1  rst=off  init_reg=0  en=off  dbl_ovrd=off  show_param=on  distributed_mem=off  use_rpm=on  gen_core=off
      settings: xl_area=[0, 0, 0, 0, 0, 0, 0]
  Register : xbsIndex_r3/Register  init=0  reg_only_valid=off  explicit_period=off  period=1  rst=off  en=off  out_en=off  dbl_ovrd=off  show_param=off
      settings: xl_area=[0, 0, 0, 0, 0, 0, 0]
  Reinterpret1 : xbsIndex_r3/Reinterpret  force_arith_type=on  arith_type=Unsigned  force_bin_pt=on  bin_pt=0  force_valid=on
  Reinterpret2 : xbsIndex_r3/Reinterpret  force_arith_type=on  arith_type=Unsigned  force_bin_pt=on  bin_pt=0  force_valid=on
  dout : Outport
  sync_out : Outport  Port=2
  coeff : Outport  Port=3
  wires:
  din/1 -> Delay1/1
  Delay1/1 -> dout/1
  sync/1 -> Counter/1, Delay/1
  Delay/1 -> sync_out/1
  Concat/1 -> Register/1
  Register/1 -> coeff/1
  Counter/1 -> ROM1/1, ROM2/1
  ROM1/1 -> Reinterpret1/1
  Reinterpret1/1 -> Concat/1
  ROM2/1 -> Reinterpret2/1
  Reinterpret2/1 -> Concat/2

== system dual500MHzPFB/cfgspec/PFB_Subsystem/pfb_fir_real/pol1_in4_last_tap/pfb_real_add_tree ==
  din : Inport  Port=1  LatchInput=off
  sync : Inport  Port=2  LatchInput=off
  Reint0 : xbsIndex_r3/Reinterpret  force_arith_type=on  arith_type="Signed  (2's comp)"  force_bin_pt=on  bin_pt=CoeffBitWidth + BitWidthIn - 2  force_valid=on
  Reint1 : xbsIndex_r3/Reinterpret  force_arith_type=on  arith_type="Signed  (2's comp)"  force_bin_pt=on  bin_pt=CoeffBitWidth + BitWidthIn - 2  force_valid=on
  Slice0 : xbsIndex_r3/Slice  mode=Upper Bit Location + Width  nbits=CoeffBitWidth + BitWidthIn  bit1=-0*(CoeffBitWidth + BitWidthIn)  base1=MSB of Input  bit0=0  base0=MSB of Input  boolean_output=off  explicit_period=off  period=1  dbl_ovrd=off
  Slice1 : xbsIndex_r3/Slice  mode=Upper Bit Location + Width  nbits=CoeffBitWidth + BitWidthIn  bit1=-1*(CoeffBitWidth + BitWidthIn)  base1=MSB of Input  bit0=0  base0=MSB of Input  boolean_output=off  explicit_period=off  period=1  dbl_ovrd=off
  adder_tree1 : Subsystem  AncestorBlock=casper_library/Misc/adder_tree  mask(adder_tree){n_inputs=2, latency=2}
      mask prompts: n_inputs "Number of Inputs"; latency "Add Latency"
      mask help: Sums all inputs using a tree of adds and delays.
      mask init:
      | adder_tree_init(gcb, ...
      |     'n_inputs', n_inputs, ...
      |     'latency', latency);
      settings: AttributesFormatString=latency 2
      mask Help: eval('xlWeb([getenv(''MLIB_ROOT''), ''\doc\html\sp_adder_tree\sp_adder_tree.html''])')
  convert1 : xbsIndex_r3/Convert  arith_type="Signed  (2's comp)"  n_bits=BitWidthOut  bin_pt=BitWidthOut-1  quantization=Truncate  overflow=Saturate  latency=add_latency  explicit_period=off  period=1  dbl_ovrd=off  show_param=off  inserted_by_tool=off  pipeline=off
      settings: xl_area=[0, 0, 0, 0, 0, 0, 0]
  delay1 : xbsIndex_r3/Delay  latency=2  reg_retiming=off  explicit_period=off  period=1  en=off  accept_only_valid=off  init_zero=on  dbl_ovrd=off  show_param=off
      settings: xl_area=[0, 0, 0, 0, 0, 0, 0]
  scale1 : xbsIndex_r3/Scale  scale_factor=-2  explicit_period=off  period=1  dbl_ovrd=off
  dout : Outport
  sync_out : Outport  Port=2
  wires:
  adder_tree1/2(dout) -> scale1/1
  scale1/1 -> convert1/1
  convert1/1 -> dout/1
  sync/1 -> adder_tree1/1(sync)
  adder_tree1/1(sync_out) -> delay1/1
  delay1/1 -> sync_out/1
  din/1 -> Slice0/1, Slice1/1
  Slice0/1 -> Reint0/1
  Reint0/1 -> adder_tree1/2(din1)
  Slice1/1 -> Reint1/1
  Reint1/1 -> adder_tree1/3(din2)

== system dual500MHzPFB/cfgspec/PFB_Subsystem/pfb_fir_real1/pol1_in1_first_tap/delay ==
  In1 : Inport  Port=1  LatchInput=off
  delay_bram : casper_library/Delays/delay_bram  DelayLen=2^(PFBSize-n_inputs)  bram_latency=bram_latency
  Out1 : Outport
  wires:
  In1/1 -> delay_bram/1
  delay_bram/1 -> Out1/1
